simulink model "pseudorange_measurement_model"  (R2016b)
settings: Solver=VariableStepAuto  StartTime=0.0  StopTime=10.0  RelTol=1e-3
settings Model: Creator=liana  LastModifiedBy=liana

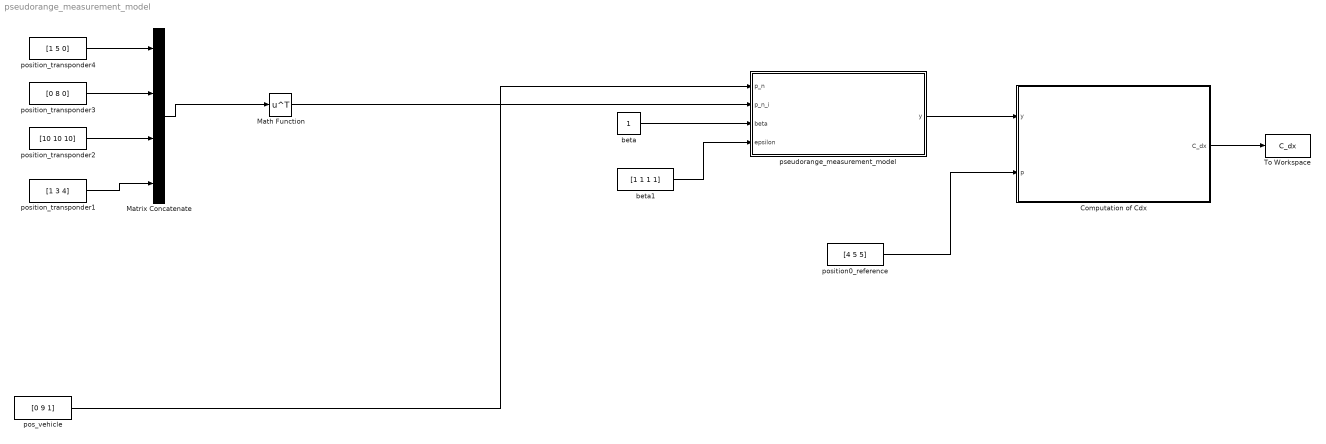
== system pseudorange_measurement_model ==
  Computation of Cdx : MATLAB Function  TreatAsAtomicUnit=on
  Math Function : Math  Operator=transpose  SaturateOnIntegerOverflow=on
  Matrix Concatenate : Concatenate  NumInputs=4  Mode=Multidimensional array  ConcatenateDimension=2
  To Workspace : ToWorkspace  VariableName=C_dx  SampleTime=-1
  beta : Constant
  beta1 : Constant  Value=[1 1 1 1]
  pos_vehicle : Constant  Value=[0 9 1]
  position0_reference : Constant  Value=[4 5 5]
  position_transponder1 : Constant  Value=[1 3 4]
  position_transponder2 : Constant  Value=[10 10 10]
  position_transponder3 : Constant  Value=[0 8 0]
  position_transponder4 : Constant  Value=[1 5 0]
  pseudorange_measurement_model : MATLAB Function  TreatAsAtomicUnit=on
  wires:
  pos_vehicle/1 -> pseudorange_measurement_model/1(p_n)
  beta/1 -> pseudorange_measurement_model/3(beta)
  beta1/1 -> pseudorange_measurement_model/4(epsilon)
  position_transponder4/1 -> Matrix Concatenate/1
  position_transponder3/1 -> Matrix Concatenate/2
  position_transponder2/1 -> Matrix Concatenate/3
  position_transponder1/1 -> Matrix Concatenate/4
  Matrix Concatenate/1 -> Math Function/1
  Math Function/1 -> pseudorange_measurement_model/2(p_n_i)
  pseudorange_measurement_model/1(y) -> Computation of Cdx/1(y)
  position0_reference/1 -> Computation of Cdx/2(p)
  Computation of Cdx/1(C_dx) -> To Workspace/1

== matlab function pseudorange_measurement_model/Computation of Cdx ==
  data: y input; p input; C_dx output size=[3,4]
function C_dx  = C_dx_func(y,p)

    % y vector 
    % p matrix has row vectors
    %            (x,y,z) cols 
    %            m-rows are transponders number
    % all variables are in navigation frame oh yeah! baby ;)
    
    [row,col] = size(p);
    [row_,col_] = size(y);
    
    % m-measure vector
    p_m = p(row,:);
    y_m = y(row_);

    m = row; % m is transpoders number
    
    
    p_ = zeros(m,3);
    y_ = zeros(m,1);
    
    for i = 1 : 1 : m-1
    
        p_(i) = p_m - p(i,:);
        y_(i) = y(i) - y_m;
        
    end
    
    C_dx = [p_, y_];

end

== matlab function pseudorange_measurement_model/pseudorange_measurement_model ==
  data: p_n input; y output size=4; p_n_i input; beta input; epsilon input
function y = pseudorange_mea_model(p_n,p_n_i,beta,epsilon)

  %  row-vector


  y = zeros(size(p_n_i,1),1);

  for i = 1: size(p_n_i,1)

      rho = norm(p_n-p_n_i(i,:)');  % eq. 7
      
      y(i) = rho + beta + epsilon(i); % eq. 8 

  end
      
end
